simulink library "pixhawk_slib_phm"  (R2017b)
settings: Solver=ode45  StartTime=0.0  StopTime=10.0  RelTol=1e-3
undefined symbols (not defined in the file or in its folder): BatteryFault, Earth, F, FaultParamAPI, Light, LoadFault, MIL, ModelParam_envAltitude, ModelParam_noiseGPSSampTime, ModelParam_noiseLowPassFilterCoeAccel, ModelParam_noiseLowPassFilterCoeGyro, ModelParam_noisePowerIMU, ModelParam_timeSampBaro, Moderate, MotorFault1, PropFault, SensorFault, WGS84, WindFault
libraries: aerolibwind2 x4, aerolibtransform2 x1, simulink x1, aerolibasang x1, aerolibatmos2 x1, aerolibnav x1, aerolibgravity2 x1
(part 1 of 2)
settings Model: Creator=skuznick  LastModifiedBy=uavcs
settings DataIOCC: LimitDataPoints=on  SaveFormat=Array
settings OptimizationCC: BlockReduction=off  BooleanDataType=off  LifeSpan=inf
settings DebuggingCC: SaveWithParameterizedLinksMsg=none  UnderspecifiedInitializationDetection=Classic  MergeDetectMultiDrivingBlocksExec=none  SignalResolutionControl=TryResolveAllWithWarning  AllowSymbolicDim=off  StrictBusMsg=Warning  SFUnexpectedBacktrackingDiag=warning  SFNoUnconditionalDefaultTransitionDiag=warning  SFExecutionAtInitializationDiag=none
settings HardwareCC: ProdBitPerPointer=32  ProdBitPerSizeT=32  ProdBitPerPtrDiffT=32  ProdLargestAtomicFloat=None  ProdIntDivRoundTo=Undefined  ProdEndianess=Unspecified  ProdWordSize=32  ProdHWDeviceType=32-bit Generic  TargetUnknown=on
settings ModelReferenceCC: PropagateSignalLabelsOutOfModel=off
settings CodeAppCC: StateflowObjectComments=on
settings GRTTargetCC: TargetLangStandard=C89/C90 (ANSI)  GeneratePreprocessorConditionals=Disable all
settings ConfigComp: CovMetricSettings=dw  CovHtmlReporting=on  CovSaveCumulativeToWorkspaceVar=on  CovSaveSingleToWorkspaceVar=on  CovExternalEMLEnable=off  CovSFcnEnable=off

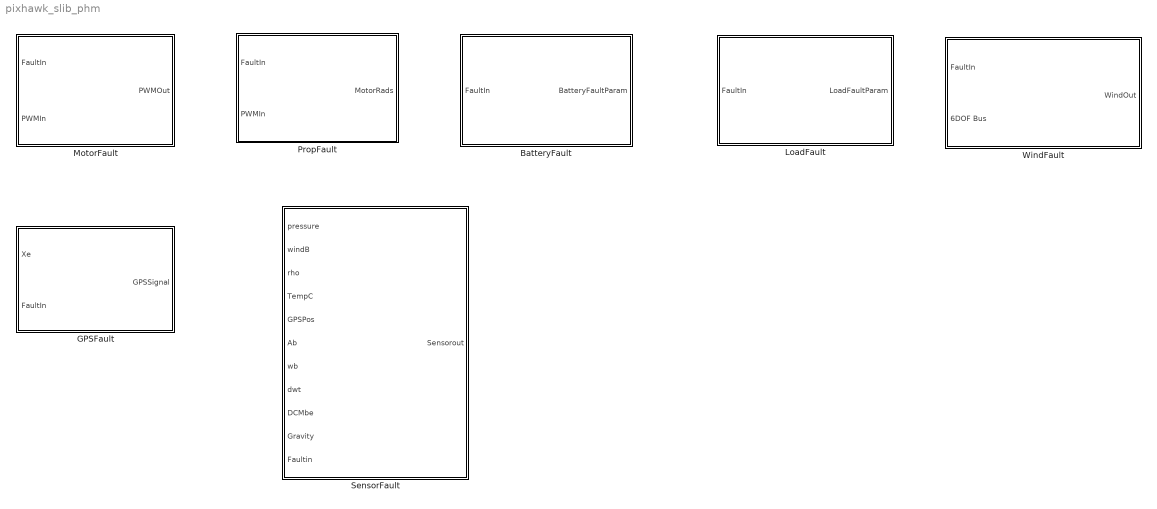
== system pixhawk_slib_phm ==
  BatteryFault : Subsystem  mask{FaultParamStruct=BatteryFault}
      mask prompts: FaultParamStruct "Fault Param Struct"
      mask Help: eval('sharedhelp(''BatteryFault'')');
  GPSFault : Subsystem  mask{FaultParamStruct=SensorFault, ComParamVect=FaultParamAPI}
      mask prompts: FaultParamStruct "Fault Param Struct"; ComParamVect "Common Param Vect"
      mask Help: eval('sharedhelp(''GPSFault'')');
      mask DialogControl ParameterGroupVar Prompt: 参数
  LoadFault : Subsystem  mask{FaultParamStruct=LoadFault}
      mask prompts: FaultParamStruct "Fault Param Struct"
      mask Help: eval('sharedhelp(''LoadFault'')');
  MotorFault : Subsystem  mask{FaultParamStruct=MotorFault1, ComParamVect=FaultParamAPI}
      mask prompts: FaultParamStruct "Fault Param Struct"; ComParamVect "Common Param Vect"
      mask Help: eval('sharedhelp(''MotorFault'')');
  PropFault : Subsystem  mask{FaultParamStruct=PropFault, ComParamVect=FaultParamAPI}
      mask prompts: FaultParamStruct "Fault Param Struct"; ComParamVect "Common Struct Vect"
      mask Help: eval('sharedhelp(''PropFault'')');
  SensorFault : Subsystem  mask{FaultParamStruct=SensorFault, ComParamVect=FaultParamAPI}
      mask prompts: FaultParamStruct "Fault Param Struct"; ComParamVect "Common Param Vect"
      mask Help: eval('sharedhelp(''SensorFault'')');
  WindFault : Subsystem  mask{FaultParamStruct=WindFault, ComParamVect=FaultParamAPI}
      mask prompts: FaultParamStruct "Fault Param Struct"; ComParamVect "Common Param Vect"
      mask Help: eval('sharedhelp(''WindFault'')');

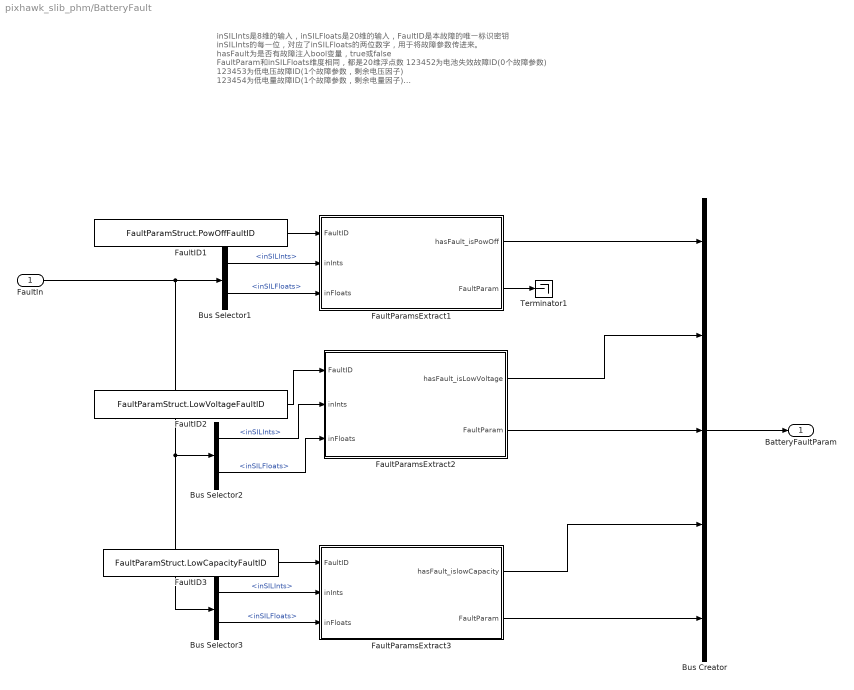
== system pixhawk_slib_phm/BatteryFault ==
  note: inSILInts是8维的输入，inSILFloats是20维的输入，FaultID是本故障的唯一标识密钥
      | inSILInts的每一位，对应了inSILFloats的两位数字，用于将故障参数传进来。
      |
      | hasFault为是否有故障注入bool变量，true或false
      | FaultParam和inSILFloats维度相同，都是20维浮点数
      |
      | 123452为电池失效故障ID(0个故障参数)
      | 123453为低电压故障ID(1个故障参数，剩余电压因子)
      | 123454为低电量故障ID(1个故障参数，剩余电量因子)
      |
      | 注：如果没有新的故障注入进来，FaultParamsExtract会保持上一时刻的值。
  FaultIn : Inport
  Bus Creator : BusCreator  Inputs=5
  Bus Selector1 : BusSelector  OutputSignals=inSILInts,inSILFloats
  Bus Selector2 : BusSelector  OutputSignals=inSILInts,inSILFloats
  Bus Selector3 : BusSelector  OutputSignals=inSILInts,inSILFloats
  FaultID1 : Constant  Value=FaultParamStruct.PowOffFaultID  OutDataTypeStr=int32
  FaultID2 : Constant  Value=FaultParamStruct.LowVoltageFaultID  OutDataTypeStr=int32
  FaultID3 : Constant  Value=FaultParamStruct.LowCapacityFaultID  OutDataTypeStr=int32
  FaultParamsExtract1 : MATLAB Function  TreatAsAtomicUnit=on
  FaultParamsExtract2 : MATLAB Function  TreatAsAtomicUnit=on
  FaultParamsExtract3 : MATLAB Function  TreatAsAtomicUnit=on
  Terminator1 : Terminator
  BatteryFaultParam : Outport  VectorParamsAs1DForOutWhenUnconnected=on
  wires:
  Bus Selector3/2 -> FaultParamsExtract3/3(inFloats)  "<inSILFloats>"
  Bus Selector3/1 -> FaultParamsExtract3/2(inInts)  "<inSILInts>"
  FaultIn/1 -> Bus Selector3/1, Bus Selector2/1, Bus Selector1/1
  Bus Selector1/1 -> FaultParamsExtract1/2(inInts)  "<inSILInts>"
  Bus Selector2/1 -> FaultParamsExtract2/2(inInts)  "<inSILInts>"
  FaultParamsExtract2/2(FaultParam) -> Bus Creator/3
  FaultID2/1 -> FaultParamsExtract2/1(FaultID)
  Bus Selector1/2 -> FaultParamsExtract1/3(inFloats)  "<inSILFloats>"
  FaultID1/1 -> FaultParamsExtract1/1(FaultID)
  FaultID3/1 -> FaultParamsExtract3/1(FaultID)
  Bus Selector2/2 -> FaultParamsExtract2/3(inFloats)  "<inSILFloats>"
  FaultParamsExtract1/2(FaultParam) -> Terminator1/1
  FaultParamsExtract1/1(hasFault_isPowOff) -> Bus Creator/1
  FaultParamsExtract2/1(hasFault_isLowVoltage) -> Bus Creator/2
  Bus Creator/1 -> BatteryFaultParam/1
  FaultParamsExtract3/1(hasFault_islowCapacity) -> Bus Creator/4
  FaultParamsExtract3/2(FaultParam) -> Bus Creator/5

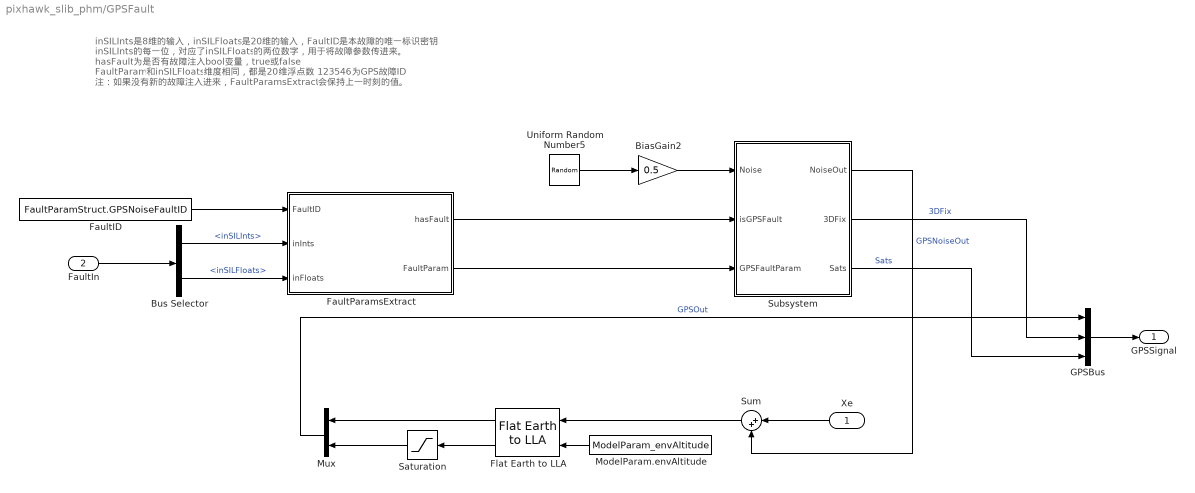
== system pixhawk_slib_phm/GPSFault ==
  note: inSILInts是8维的输入，inSILFloats是20维的输入，FaultID是本故障的唯一标识密钥
      | inSILInts的每一位，对应了inSILFloats的两位数字，用于将故障参数传进来。
      |
      | hasFault为是否有故障注入bool变量，true或false
      | FaultParam和inSILFloats维度相同，都是20维浮点数
      |
      | 123546为GPS故障ID
      |
      | 注：如果没有新的故障注入进来，FaultParamsExtract会保持上一时刻的值。
  Xe : Inport
  FaultIn : Inport  Port=2
  BiasGain2 : Gain  Gain=0.5
  Bus Selector : BusSelector  OutputSignals=inSILInts,inSILFloats
  FaultID : Constant  Value=FaultParamStruct.GPSNoiseFaultID  OutDataTypeStr=int32
  FaultParamsExtract : MATLAB Function  TreatAsAtomicUnit=on
  Flat Earth to LLA : aerolibtransform2/Flat Earth to LLA  units=Metric (MKS)  ptype=Earth (WGS84)  F=1/298.257223563  R=6378137  LL0=ModelParam_GPSLatLong  psi=0
  GPSBus : BusCreator  Inputs=3
  ModelParam.envAltitude : Constant  Value=ModelParam_envAltitude
  Mux : Mux  Inputs=2
  Saturation : Saturate  UpperLimit=100000  LowerLimit=0
  Subsystem : Subsystem
  Sum : Sum  Inputs=|++
  Uniform Random Number5 : UniformRandomNumber  Minimum=[-1,-1,-2]  Maximum=[1,1,2]  Seed=[1452,787,69]  SampleTime=ModelParam_noiseGPSSampTime
  GPSSignal : Outport  VectorParamsAs1DForOutWhenUnconnected=on
  wires:
  FaultParamsExtract/1(hasFault) -> Subsystem/2(isGPSFault)
  FaultParamsExtract/2(FaultParam) -> Subsystem/3(GPSFaultParam)
  Subsystem/3(Sats) -> GPSBus/3  "Sats"
  Saturation/1 -> Mux/2
  Flat Earth to LLA/2 -> Saturation/1
  Uniform Random Number5/1 -> BiasGain2/1
  FaultID/1 -> FaultParamsExtract/1(FaultID)
  BiasGain2/1 -> Subsystem/1(Noise)
  Bus Selector/1 -> FaultParamsExtract/2(inInts)  "<inSILInts>"
  FaultIn/1 -> Bus Selector/1
  Flat Earth to LLA/1 -> Mux/1
  Xe/1 -> Sum/1
  GPSBus/1 -> GPSSignal/1
  Subsystem/2(3DFix) -> GPSBus/2  "3DFix"
  ModelParam.envAltitude/1 -> Flat Earth to LLA/2
  Mux/1 -> GPSBus/1  "GPSOut"
  Subsystem/1(NoiseOut) -> Sum/2  "GPSNoiseOut"
  Bus Selector/2 -> FaultParamsExtract/3(inFloats)  "<inSILFloats>"
  Sum/1 -> Flat Earth to LLA/1

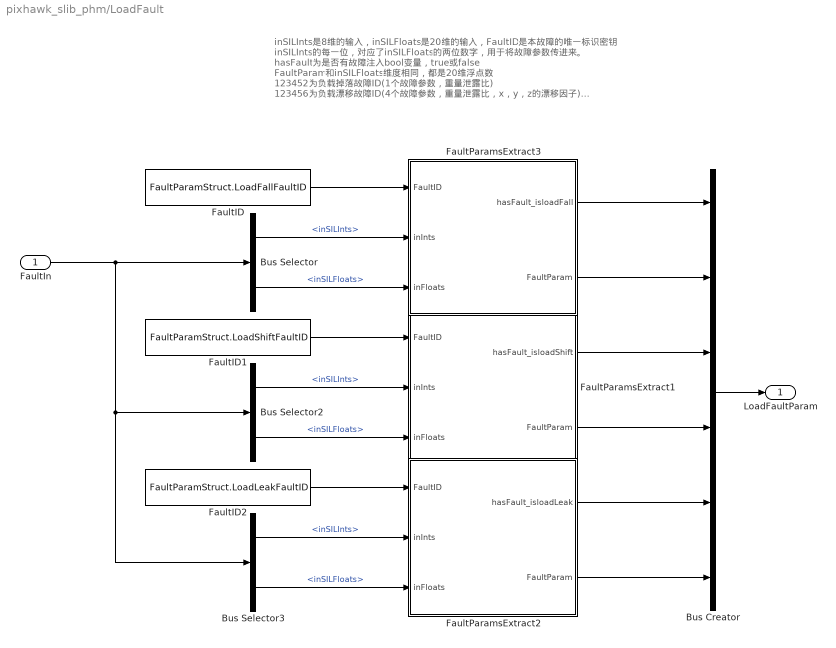
== system pixhawk_slib_phm/LoadFault ==
  note: inSILInts是8维的输入，inSILFloats是20维的输入，FaultID是本故障的唯一标识密钥
      | inSILInts的每一位，对应了inSILFloats的两位数字，用于将故障参数传进来。
      |
      | hasFault为是否有故障注入bool变量，true或false
      | FaultParam和inSILFloats维度相同，都是20维浮点数
      |
      | 123452为负载掉落故障ID(1个故障参数，重量泄露比)
      | 123456为负载漂移故障ID(4个故障参数，重量泄露比，x，y，z的漂移因子)
      | 123457为负载泄露故障ID(2个故障参数，1个重量泄露比，1个泄露因子)
      | 注：如果没有新的故障注入进来，FaultParamsExtract会保持上一时刻的值。
  FaultIn : Inport
  Bus Creator : BusCreator  Inputs=6
  Bus Selector : BusSelector  OutputSignals=inSILInts,inSILFloats
  Bus Selector2 : BusSelector  OutputSignals=inSILInts,inSILFloats
  Bus Selector3 : BusSelector  OutputSignals=inSILInts,inSILFloats
  FaultID : Constant  Value=FaultParamStruct.LoadFallFaultID  OutDataTypeStr=int32
  FaultID1 : Constant  Value=FaultParamStruct.LoadShiftFaultID  OutDataTypeStr=int32
  FaultID2 : Constant  Value=FaultParamStruct.LoadLeakFaultID  OutDataTypeStr=int32
  FaultParamsExtract1 : MATLAB Function  TreatAsAtomicUnit=on
  FaultParamsExtract2 : MATLAB Function  TreatAsAtomicUnit=on
  FaultParamsExtract3 : MATLAB Function  TreatAsAtomicUnit=on
  LoadFaultParam : Outport  VectorParamsAs1DForOutWhenUnconnected=on
  wires:
  FaultIn/1 -> Bus Selector3/1, Bus Selector2/1, Bus Selector/1
  Bus Selector3/2 -> FaultParamsExtract2/3(inFloats)  "<inSILFloats>"
  Bus Selector/1 -> FaultParamsExtract3/2(inInts)  "<inSILInts>"
  Bus Selector2/2 -> FaultParamsExtract1/3(inFloats)  "<inSILFloats>"
  Bus Selector3/1 -> FaultParamsExtract2/2(inInts)  "<inSILInts>"
  Bus Selector2/1 -> FaultParamsExtract1/2(inInts)  "<inSILInts>"
  Bus Selector/2 -> FaultParamsExtract3/3(inFloats)  "<inSILFloats>"
  FaultID/1 -> FaultParamsExtract3/1(FaultID)
  FaultID2/1 -> FaultParamsExtract2/1(FaultID)
  FaultID1/1 -> FaultParamsExtract1/1(FaultID)
  FaultParamsExtract3/1(hasFault_isloadFall) -> Bus Creator/1
  FaultParamsExtract3/2(FaultParam) -> Bus Creator/2
  FaultParamsExtract1/1(hasFault_isloadShift) -> Bus Creator/3
  FaultParamsExtract1/2(FaultParam) -> Bus Creator/4
  FaultParamsExtract2/1(hasFault_isloadLeak) -> Bus Creator/5
  FaultParamsExtract2/2(FaultParam) -> Bus Creator/6
  Bus Creator/1 -> LoadFaultParam/1

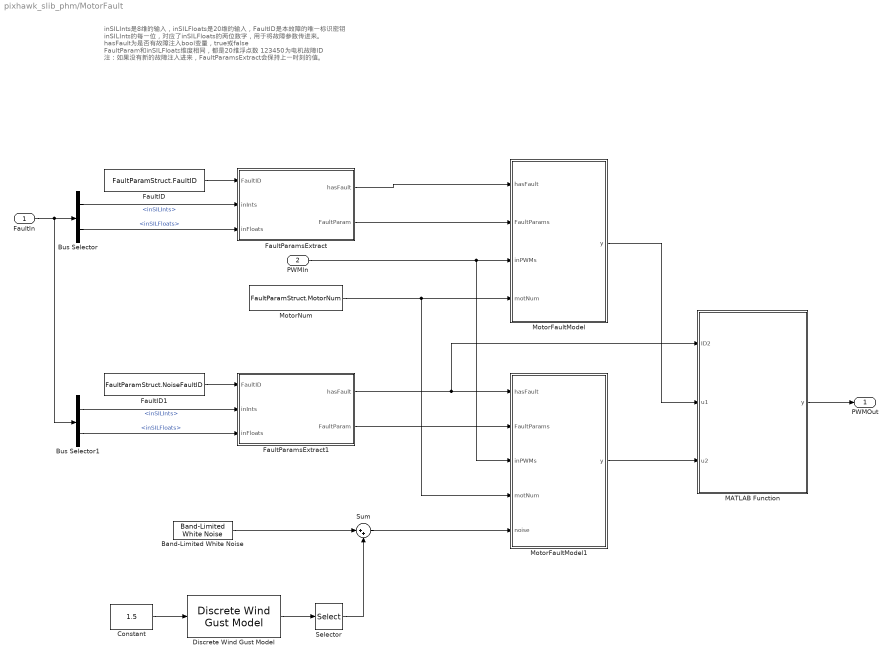
== system pixhawk_slib_phm/MotorFault ==
  note: inSILInts是8维的输入，inSILFloats是20维的输入，FaultID是本故障的唯一标识密钥
      | inSILInts的每一位，对应了inSILFloats的两位数字，用于将故障参数传进来。
      |
      | hasFault为是否有故障注入bool变量，true或false
      | FaultParam和inSILFloats维度相同，都是20维浮点数
      |
      | 123450为电机故障ID
      |
      | 注：如果没有新的故障注入进来，FaultParamsExtract会保持上一时刻的值。
  FaultIn : Inport
  PWMIn : Inport  Port=2
  Band-Limited White Noise : simulink/Sources/Band-Limited White Noise  Cov=[1]  Ts=0.1  seed=[23341]
  Bus Selector : BusSelector  OutputSignals=inSILInts,inSILFloats
  Bus Selector1 : BusSelector  OutputSignals=inSILInts,inSILFloats
  Constant : Constant  Value=1.5
  Discrete Wind Gust Model : aerolibwind2/Discrete Wind Gust Model  units=Metric (MKS)  Gx=on  Gy=on  Gz=on  t_0=ComParamVect.FaultInParams(3)  d_m=[120 120 80]  v_m=[3.5 3.5 3.0]
  FaultID : Constant  Value=FaultParamStruct.FaultID  OutDataTypeStr=int32
  FaultID1 : Constant  Value=FaultParamStruct.NoiseFaultID  OutDataTypeStr=int32
  FaultParamsExtract : MATLAB Function  TreatAsAtomicUnit=on
  FaultParamsExtract1 : MATLAB Function  TreatAsAtomicUnit=on
  MATLAB Function : MATLAB Function  TreatAsAtomicUnit=on
  MotorFaultModel : MATLAB Function  TreatAsAtomicUnit=on
  MotorFaultModel1 : MATLAB Function  TreatAsAtomicUnit=on
  MotorNum : Constant  Value=FaultParamStruct.MotorNum  OutDataTypeStr=int32
  Selector : Selector  InputPortWidth=3  IndexOptions=Index vector (dialog)  Indices=[1]  OutputSizes=1
  Sum : Sum  Inputs=|++
  PWMOut : Outport  VectorParamsAs1DForOutWhenUnconnected=on
  wires:
  FaultIn/1 -> Bus Selector1/1, Bus Selector/1
  FaultParamsExtract/2(FaultParam) -> MotorFaultModel/2(FaultParams)
  FaultParamsExtract/1(hasFault) -> MotorFaultModel/1(hasFault)
  PWMIn/1 -> MotorFaultModel1/3(inPWMs), MotorFaultModel/3(inPWMs)
  FaultID/1 -> FaultParamsExtract/1(FaultID)
  MotorFaultModel/1(y) -> MATLAB Function/2(u1)
  Bus Selector/2 -> FaultParamsExtract/3(inFloats)  "<inSILFloats>"
  Constant/1 -> Discrete Wind Gust Model/1
  Selector/1 -> Sum/2
  Sum/1 -> MotorFaultModel1/5(noise)
  Discrete Wind Gust Model/1 -> Selector/1
  Band-Limited White Noise/1 -> Sum/1
  Bus Selector/1 -> FaultParamsExtract/2(inInts)  "<inSILInts>"
  MotorNum/1 -> MotorFaultModel1/4(motNum), MotorFaultModel/4(motNum)
  Bus Selector1/1 -> FaultParamsExtract1/2(inInts)  "<inSILInts>"
  Bus Selector1/2 -> FaultParamsExtract1/3(inFloats)  "<inSILFloats>"
  FaultParamsExtract1/1(hasFault) -> MATLAB Function/1(ID2), MotorFaultModel1/1(hasFault)
  FaultParamsExtract1/2(FaultParam) -> MotorFaultModel1/2(FaultParams)
  FaultID1/1 -> FaultParamsExtract1/1(FaultID)
  MotorFaultModel1/1(y) -> MATLAB Function/3(u2)
  MATLAB Function/1(y) -> PWMOut/1

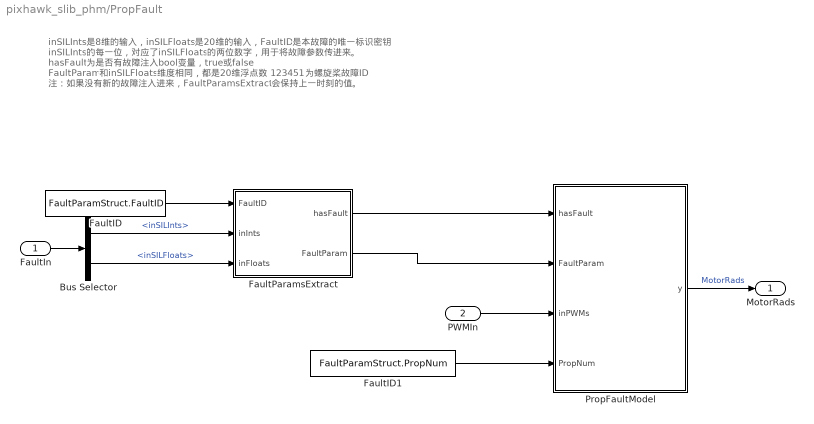
== system pixhawk_slib_phm/PropFault ==
  note: inSILInts是8维的输入，inSILFloats是20维的输入，FaultID是本故障的唯一标识密钥
      | inSILInts的每一位，对应了inSILFloats的两位数字，用于将故障参数传进来。
      |
      | hasFault为是否有故障注入bool变量，true或false
      | FaultParam和inSILFloats维度相同，都是20维浮点数
      |
      | 123451为螺旋桨故障ID
      | 注：如果没有新的故障注入进来，FaultParamsExtract会保持上一时刻的值。
  FaultIn : Inport
  PWMIn : Inport  Port=2
  Bus Selector : BusSelector  OutputSignals=inSILInts,inSILFloats
  FaultID : Constant  Value=FaultParamStruct.FaultID  OutDataTypeStr=int32
  FaultID1 : Constant  Value=FaultParamStruct.PropNum  OutDataTypeStr=int32
  FaultParamsExtract : MATLAB Function  TreatAsAtomicUnit=on
  PropFaultModel : MATLAB Function  TreatAsAtomicUnit=on
  MotorRads : Outport
  wires:
  FaultParamsExtract/1(hasFault) -> PropFaultModel/1(hasFault)
  Bus Selector/2 -> FaultParamsExtract/3(inFloats)  "<inSILFloats>"
  FaultID/1 -> FaultParamsExtract/1(FaultID)
  Bus Selector/1 -> FaultParamsExtract/2(inInts)  "<inSILInts>"
  FaultParamsExtract/2(FaultParam) -> PropFaultModel/2(FaultParam)
  PWMIn/1 -> PropFaultModel/3(inPWMs)
  PropFaultModel/1(y) -> MotorRads/1  "MotorRads"
  FaultIn/1 -> Bus Selector/1
  FaultID1/1 -> PropFaultModel/4(PropNum)

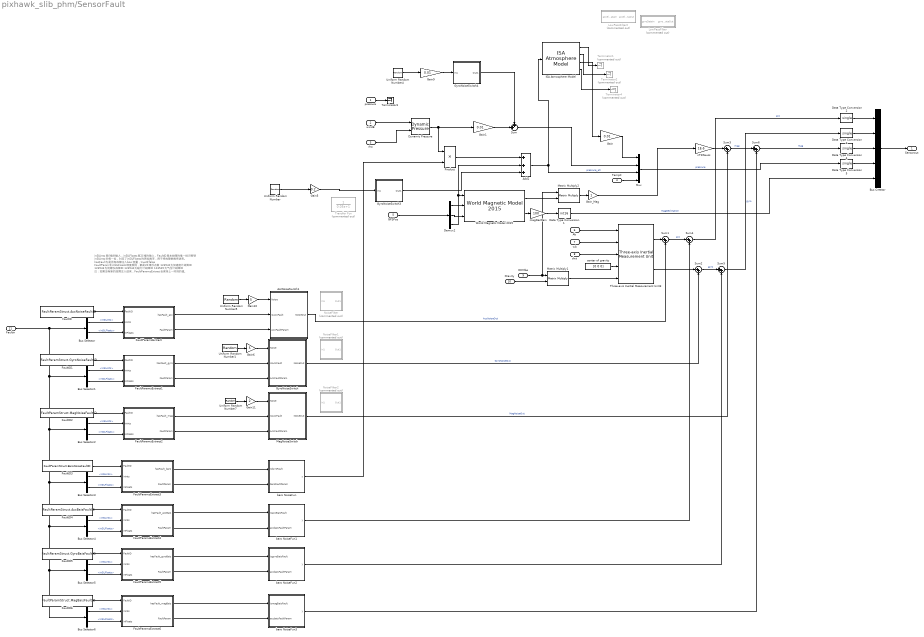
== system pixhawk_slib_phm/SensorFault ==
  note: inSILInts是8维的输入，inSILFloats是20维的输入，FaultID是本故障的唯一标识密钥
      | inSILInts的每一位，对应了inSILFloats的两位数字，用于将故障参数传进来。
      |
      | hasFault为是否有故障注入bool变量，true或false
      | FaultParam和inSILFloats维度相同，都是20维浮点数
      |
      | 123542为加速度计故障ID
      | 123543为陀螺仪故障ID
      | 123544为磁力计故障ID
      | 123545为气压计故障ID
      | 注：如果没有新的故障注入进来，FaultParamsExtract会保持上一时刻的值。
  pressure : Inport
  windB : Inport  Port=2
  rho : Inport  Port=3
  TempC : Inport  Port=4
  GPSPos : Inport  Port=5
  Ab : Inport  Port=6
  wb : Inport  Port=7
  dwt : Inport  Port=8
  DCMbe : Inport  Port=9
  Gravity : Inport  Port=10
  Faultin : Inport  Port=11
  AccNoiseSwitch1 : Subsystem
  Add2 : Sum  Inputs=+++
  Bus Creator : BusCreator  Inputs=5
  Bus Selector{,1..6} (7 alike) : BusSelector  OutputSignals=inSILInts,inSILFloats
  Data Type Conversion1 : DataTypeConversion  OutDataTypeStr=int16
  Data Type Conversion{2..5} (4 alike) : DataTypeConversion  OutDataTypeStr=single
  Demux2 : Demux  Outputs=3
  Dynamic Pressure : aerolibasang/Dynamic Pressure
  FaultID : Constant  Value=FaultParamStruct.AccNoiseFaultID  OutDataTypeStr=int32
  FaultID1 : Constant  Value=FaultParamStruct.GyroNoiseFaultID  OutDataTypeStr=int32
  FaultID2 : Constant  Value=FaultParamStruct.MagNoiseFaultID  OutDataTypeStr=int32
  FaultID3 : Constant  Value=FaultParamStruct.BaroNoiseFaultID  OutDataTypeStr=int32
  FaultID4 : Constant  Value=FaultParamStruct.AccBaisFaultID  OutDataTypeStr=int32
  FaultID5 : Constant  Value=FaultParamStruct.GyroBaisFaultID  OutDataTypeStr=int32
  FaultID6 : Constant  Value=FaultParamStruct.MagBaisFaultID  OutDataTypeStr=int32
  FaultParamsExtract : MATLAB Function  TreatAsAtomicUnit=on
  FaultParamsExtract1 : MATLAB Function  TreatAsAtomicUnit=on
  FaultParamsExtract2 : MATLAB Function  TreatAsAtomicUnit=on
  FaultParamsExtract3 : MATLAB Function  TreatAsAtomicUnit=on
  FaultParamsExtract4 : MATLAB Function  TreatAsAtomicUnit=on
  FaultParamsExtract5 : MATLAB Function  TreatAsAtomicUnit=on
  FaultParamsExtract6 : MATLAB Function  TreatAsAtomicUnit=on
  Gain : Gain  Gain=0.01
  Gain1 : Gain  Gain=0.01
  Gain10 : Gain  Gain=5
  Gain11 : Gain  Gain=2
  Gain5 : Gain  Gain=0.2
  Gain6 : Gain  Gain=5
  Gain9 : Gain  Gain=0.01
  Gain_Mag : Gain
  GyroNoiseSwitch : Subsystem
  GyroNoiseSwitch3 : Subsystem
  GyroNoiseSwitch4 : Subsystem
  ISA Atmosphere Model : aerolibatmos2/ISA Atmosphere Model  custom=off  g=9.80665  gamma=1.4  R=287.0531  L=0.0065  h_trop=11000  h_strat=20000  rho0=1.225  P0=101325  T0=288.15  h0=0
  LowPassFilter : Subsystem  Commented=on
  LowPassFilter2 : Subsystem  Commented=on
  MagNoiseSwitch : Subsystem
  Matrix Multiply1 : Product  Multiplication=Matrix(*)
  Matrix Multiply2 : Product  Multiplication=Matrix(*)
  Mux : Mux
  NoiseFilter : Subsystem  Commented=on
  NoiseFilter1 : Subsystem  Commented=on
  NoiseFilter2 : Subsystem  Commented=on
  Product : Product
  Sum : Sum  Inputs=++|
  Sum{1..6} (6 alike) : Sum  Inputs=|++
  Terminator1 : Terminator  Commented=on
  Terminator2 : Terminator  Commented=on
  Terminator3 : Terminator
  Terminator4 : Terminator  Commented=on
  Three-axis Inertial Measurement Unit3 : aerolibnav/Three-axis Inertial Measurement Unit  units=Metric (MKS)  imu=[0 0 0]  i_Ts=0  dtype_a=on  w_a=ComParamVect.FaultInParams(1)  z_a=ComParamVect.FaultInParams(2)  a_sf_cc=[1 0 0; 0 1 0; 0 0 1]  a_bias=[ComParamVect.FaultInParams(3) ComParamVect.FaultInParams(4) ComParamVect.FaultInParams(5)]  a_sat="[-160  -160  -160 160 160 160]"  dtype_g=on  w_g=ComParamVect.FaultInParams(6)  z_g=ComParamVect.FaultInParams(7)  g_sf_cc=[1 0 0; 0 1 0; 0 0 1]  g_bias=[ComParamVect.FaultInParams(8) ComParamVect.FaultInParams(9) ComParamVect.FaultInParams(10)]  g_sens=[ComParamVect.FaultInParams(11) ComParamVect.FaultInParams(12) ComParamVect.FaultInParams(13)]  g_sat="[-4.36  -4.36  -4.36 4.36 4.36 4.36]"  i_rand=off  i_seeds=[23093 23094 23095 23096 23097 23098]  i_pow=ModelParam_noisePowerIMU*[0.0000005 0.0000005 0.0000005 0.000000002 0.000000002 0.000000002]
  Transfer Fcn : TransferFcn  Commented=on  Denominator=[0.05 1]
  Uniform Random Number : UniformRandomNumber  Minimum=-2  Maximum=2  Seed=15634  SampleTime=ModelParam_timeSampBaro
  Uniform Random Number1 : UniformRandomNumber  Minimum=-[0.01,0.01,0.01]  Maximum=[0.01,0.01,0.01]  Seed=[3243,44556,2334343]  SampleTime=0.003
  Uniform Random Number4 : UniformRandomNumber  Seed=25634  SampleTime=0.01
  Uniform Random Number5 : UniformRandomNumber  Minimum=-[0.1,0.1,0.2]  Maximum=[0.1,0.1,0.2]  Seed=[12233,645554,678766]  SampleTime=0.003
  Uniform Random Number7 : UniformRandomNumber  Minimum=-[0.01,0.01,0.01]  Maximum=[0.01,0.01,0.01]  Seed=[45465,454534,1234232]  SampleTime=0.003
  World Magnetic Model 2015 : aerolibgravity2/World Magnetic Model 2015  units=Metric (MKS)  time_in=off  month=November  day=3  year=2017  action=Error  h_out=off  dec_out=on  inc_out=off  ti_out=off
      settings: SourceProductBaseCode=AE
  baro NoiseFun : MATLAB Function  TreatAsAtomicUnit=on
  baro NoiseFun1 : MATLAB Function  TreatAsAtomicUnit=on
  baro NoiseFun2 : MATLAB Function  TreatAsAtomicUnit=on
  baro NoiseFun3 : MATLAB Function  TreatAsAtomicUnit=on
  center of gravity : Constant  Value=[0 0 0]
  magDecGain : Gain  Gain=100
  nT2Gauss : Gain  Gain=1E-5
  Sensorout : Outport  VectorParamsAs1DForOutWhenUnconnected=on
  wires:
  FaultParamsExtract3/2(FaultParam) -> baro NoiseFun/2(baroFaultParam)
  Gain9/1 -> GyroNoiseSwitch4/1(In1)
  Matrix Multiply1/1 -> Three-axis Inertial Measurement Unit3/5
  Three-axis Inertial Measurement Unit3/1 -> Sum1/1
  FaultParamsExtract1/1(hasFault_gyro) -> GyroNoiseSwitch/2(isAccFault)
  FaultParamsExtract1/2(FaultParam) -> GyroNoiseSwitch/3(AccFaultParam)
  FaultParamsExtract/1(hasFault_acc) -> AccNoiseSwitch1/2(isAccFault)
  Bus Selector3/1 -> FaultParamsExtract3/2(inInts)  "<inSILInts>"
  Mux/1 -> Data Type Conversion5/1  "pressure"
  FaultID/1 -> FaultParamsExtract/1(FaultID)
  Sum/1 -> Mux/2
  Add2/1 -> ISA Atmosphere Model/1, Mux/3  "pressure_alt"
  TempC/1 -> Mux/4
  Gain11/1 -> MagNoiseSwitch/1(Noise)
  nT2Gauss/1 -> Sum3/1
  center of gravity/1 -> Three-axis Inertial Measurement Unit3/4
  Gravity/1 -> Matrix Multiply1/2
  Bus Selector1/2 -> FaultParamsExtract1/3(inFloats)  "<inSILFloats>"
  FaultID2/1 -> FaultParamsExtract2/1(FaultID)
  World Magnetic Model 2015/1 -> Matrix Multiply2/2
  Bus Selector3/2 -> FaultParamsExtract3/3(inFloats)  "<inSILFloats>"
  magDecGain/1 -> Data Type Conversion1/1
  DCMbe/1 -> Matrix Multiply2/1, Matrix Multiply1/1
  Three-axis Inertial Measurement Unit3/2 -> Sum2/1
  Gain_Mag/1 -> nT2Gauss/1
  Bus Selector1/1 -> FaultParamsExtract1/2(inInts)  "<inSILInts>"
  Gain6/1 -> GyroNoiseSwitch/1(Noise)
  ISA Atmosphere Model/3 -> Gain/1
  Gain1/1 -> Sum/2
  Bus Selector/2 -> FaultParamsExtract/3(inFloats)  "<inSILFloats>"
  FaultParamsExtract3/1(hasFault_baro) -> baro NoiseFun/1(isbyroFault)
  Uniform Random Number1/1 -> Gain6/1
  FaultID1/1 -> FaultParamsExtract1/1(FaultID)
  baro NoiseFun/1(y) -> Product/2
  GyroNoiseSwitch/1(NoiseOut) -> Sum2/2  "GyroNoiseOut"
  ISA Atmosphere Model/1 -> Terminator1/1
  Gain/1 -> Mux/1
  pressure/1 -> Terminator3/1
  Demux2/1 -> World Magnetic Model 2015/2
  Bus Selector2/1 -> FaultParamsExtract2/2(inInts)  "<inSILInts>"
  Uniform Random Number4/1 -> Gain9/1
  GyroNoiseSwitch4/1(Out1) -> Sum/1
  ISA Atmosphere Model/2 -> Terminator2/1
  windB/1 -> Dynamic Pressure/1
  FaultID3/1 -> FaultParamsExtract3/1(FaultID)
  GPSPos/1 -> Demux2/1
  Uniform Random Number/1 -> Gain5/1
  Bus Selector/1 -> FaultParamsExtract/2(inInts)  "<inSILInts>"
  dwt/1 -> Three-axis Inertial Measurement Unit3/3
  FaultParamsExtract2/2(FaultParam) -> MagNoiseSwitch/3(AccFaultParam)
  World Magnetic Model 2015/2 -> magDecGain/1
  GyroNoiseSwitch3/1(Out1) -> Add2/3
  Faultin/1 -> Bus Selector3/1, Bus Selector5/1, Bus Selector6/1, Bus Selector4/1, Bus Selector2/1, Bus Selector1/1, Bus Selector/1
  Demux2/3 -> World Magnetic Model 2015/1, Add2/2
  Bus Selector2/2 -> FaultParamsExtract2/3(inFloats)  "<inSILFloats>"
  MagNoiseSwitch/1(NoiseOut) -> Sum3/2  "MagNoiseOut"
  Gain10/1 -> AccNoiseSwitch1/1(Noise)
  Dynamic Pressure/1 -> Gain1/1, Product/1
  Uniform Random Number7/1 -> Gain11/1
  Matrix Multiply2/1 -> Gain_Mag/1
  Uniform Random Number5/1 -> Gain10/1
  Product/1 -> Add2/1
  ISA Atmosphere Model/4 -> Terminator4/1
  FaultParamsExtract2/1(hasFault_mag) -> MagNoiseSwitch/2(isAccFault)
  Gain5/1 -> GyroNoiseSwitch3/1(In1)
  Demux2/2 -> World Magnetic Model 2015/3
  FaultParamsExtract/2(FaultParam) -> AccNoiseSwitch1/3(AccFaultParam)
  rho/1 -> Dynamic Pressure/2
  Data Type Conversion1/1 -> Bus Creator/5  "MagDeclination"
  Bus Creator/1 -> Sensorout/1
  Data Type Conversion2/1 -> Bus Creator/1
  Data Type Conversion3/1 -> Bus Creator/2
  Data Type Conversion4/1 -> Bus Creator/3
  Data Type Conversion5/1 -> Bus Creator/4
  Ab/1 -> Three-axis Inertial Measurement Unit3/1
  wb/1 -> Three-axis Inertial Measurement Unit3/2
  AccNoiseSwitch1/1(NoiseOut) -> Sum1/2  "AccNoiseOut"
  FaultID4/1 -> FaultParamsExtract4/1(FaultID)
  Bus Selector4/1 -> FaultParamsExtract4/2(inInts)  "<inSILInts>"
  Bus Selector4/2 -> FaultParamsExtract4/3(inFloats)  "<inSILFloats>"
  FaultParamsExtract4/1(hasFault_accBais) -> baro NoiseFun1/1(isaccBaisFault)
  FaultParamsExtract4/2(FaultParam) -> baro NoiseFun1/2(accbaisFaultParam)
  Sum1/1 -> Sum4/1  "acc"
  Sum4/1 -> Data Type Conversion2/1  "acc"
  baro NoiseFun1/1(y) -> Sum4/2
  FaultParamsExtract5/1(hasFault_gyroBais) -> baro NoiseFun2/1(isgyroBaisFault)
  Bus Selector5/2 -> FaultParamsExtract5/3(inFloats)  "<inSILFloats>"
  Bus Selector5/1 -> FaultParamsExtract5/2(inInts)  "<inSILInts>"
  FaultID5/1 -> FaultParamsExtract5/1(FaultID)
  FaultParamsExtract5/2(FaultParam) -> baro NoiseFun2/2(accbaisFaultParam)
  FaultID6/1 -> FaultParamsExtract6/1(FaultID)
  FaultParamsExtract6/2(FaultParam) -> baro NoiseFun3/2(accbaisFaultParam)
  Bus Selector6/2 -> FaultParamsExtract6/3(inFloats)  "<inSILFloats>"
  FaultParamsExtract6/1(hasFault_magBais) -> baro NoiseFun3/1(ismagBaisFault)
  Bus Selector6/1 -> FaultParamsExtract6/2(inInts)  "<inSILInts>"
  Sum2/1 -> Sum5/1  "gyro"
  Sum5/1 -> Data Type Conversion3/1  "gyro"
  baro NoiseFun2/1(y) -> Sum5/2
  Sum3/1 -> Sum6/1  "mag"
  baro NoiseFun3/1(y) -> Sum6/2
  Sum6/1 -> Data Type Conversion4/1  "mag"

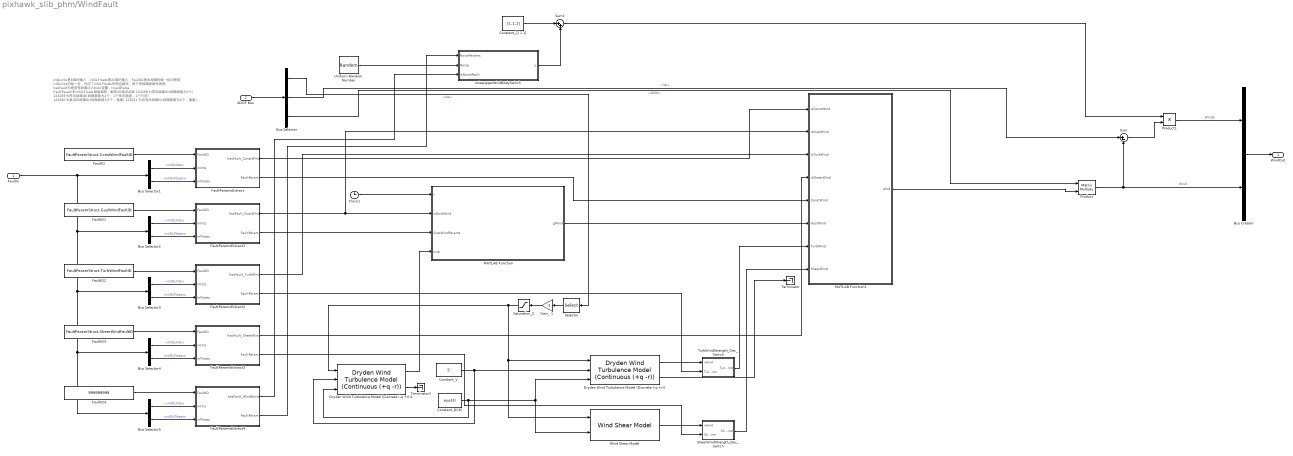
== system pixhawk_slib_phm/WindFault ==
  note: inSILInts是8维的输入，inSILFloats是20维的输入，FaultID是本故障的唯一标识密钥
      | inSILInts的每一位，对应了inSILFloats的两位数字，用于将故障参数传进来。
      |
      | hasFault为是否有故障注入bool变量，true或false
      | FaultParam和inSILFloats维度相同，都是20维浮点数
      |
      | 123458为常风故障ID(故障参数为3个)
      | 123459为阵风故障ID(故障参数为2个，1个阵风强度，1个方向)
      | 123540为紊流风故障ID(故障参数为1个，强度)
      | 123541为切向风故障ID(故障参数为1个，强度)
      |
      | 注：如果没有新的故障注入进来，FaultParamsExtract会保持上一时刻的值。
  FaultIn : Inport
  6DOF Bus : Inport  Port=2
  Bus Creator : BusCreator  Inputs=2
  Bus Selector : BusSelector  OutputSignals=Xe,Vb,DCM
  Bus Selector{1..5} (5 alike) : BusSelector  OutputSignals=inSILInts,inSILFloats
  Clock1 : Clock
  Constant_DCM : Constant  Value=eye(3)
  Constant_V : Constant  Value=5
  Constant_[1 1 1] : Constant  Value=[1,1,1]  VectorParams1D=off
  Dryden Wind Turbulence Model (Discrete (-q +r)) : aerolibwind2/Dryden Wind Turbulence Model  (Continuous (+q -r))  units=Metric (MKS)  spec=MIL-F-8785C  model=Discrete Dryden (-q +r)  W20=3  Wdeg=1  TurbProb=10^-3 - Moderate  L_high=533.4  Wingspan=1  ts=ModelParam_timeSampTurbWind  Seed=[23341 23342 23343 23344]  T_on=on
  Dryden Wind Turbulence Model (Discrete (-q +r))1 : aerolibwind2/Dryden Wind Turbulence Model  (Continuous (+q -r))  units=Metric (MKS)  spec=MIL-F-8785C  model=Discrete Dryden (-q +r)  W20=2  Wdeg=1  TurbProb=10^-2 - Light  L_high=533.4  Wingspan=1  ts=ModelParam_timeSampTurbWind  Seed=[23301 23542 82443 33344]  T_on=on
  FaultID : Constant  Value=FaultParamStruct.ConstWindFaultID  OutDataTypeStr=int32
  FaultID1 : Constant  Value=FaultParamStruct.GustWindFaultID  OutDataTypeStr=int32
  FaultID2 : Constant  Value=FaultParamStruct.TurbWindFaultID  OutDataTypeStr=int32
  FaultID3 : Constant  Value=FaultParamStruct.SheerWindFaultID  OutDataTypeStr=int32
  FaultID4 : Constant  Value=999999999  OutDataTypeStr=int32
  FaultParamsExtract : MATLAB Function  TreatAsAtomicUnit=on
  FaultParamsExtract1 : MATLAB Function  TreatAsAtomicUnit=on
  FaultParamsExtract2 : MATLAB Function  TreatAsAtomicUnit=on
  FaultParamsExtract3 : MATLAB Function  TreatAsAtomicUnit=on
  FaultParamsExtract4 : MATLAB Function  TreatAsAtomicUnit=on
  Gain_-1 : Gain  Gain=-1
  MATLAB Function : MATLAB Function  TreatAsAtomicUnit=on
  MATLAB Function1 : MATLAB Function  TreatAsAtomicUnit=on
  Product : Product  Multiplication=Matrix(*)
  Product1 : Product
  Saturation_2 : Saturate  UpperLimit=10000  LowerLimit=0
  Selector : Selector  InputPortWidth=3  IndexOptions=Index vector (dialog)  Indices=[3]  OutputSizes=1
  SheerWindStrength_Dec_Switch : MATLAB Function  TreatAsAtomicUnit=on
  Sum : Sum  Inputs=|+-
  Sum1 : Sum  Inputs=|++
  Terminator : Terminator
  Terminator1 : Terminator
  TurbWindStrength_Dec_Switch : MATLAB Function  TreatAsAtomicUnit=on
  Uniform Random Number : UniformRandomNumber  Minimum=[-1,-1,-0.5]  Maximum=[1,1,0.5]  Seed=[564565,6846798,46545]  SampleTime=0.003
  Wind Shear Model : aerolibwind2/Wind Shear Model  units=Metric (MKS)  phase=Category C - Terminal Flight Phase  W_20=3  Wdeg=1
  noiseUpperWindBodySwitch : MATLAB Function  TreatAsAtomicUnit=on
  WindOut : Outport  VectorParamsAs1DForOutWhenUnconnected=on
  wires:
  Product/1 -> Bus Creator/2, Sum/2  "Wind"
  Constant_DCM/1 -> Dryden Wind Turbulence Model (Discrete (-q +r))/3, Wind Shear Model/2, Dryden Wind Turbulence Model (Discrete (-q +r))1/3
  Clock1/1 -> MATLAB Function/1(t)
  FaultParamsExtract2/2(FaultParam) -> TurbWindStrength_Dec_Switch/2(TurbWindParams)
  FaultID1/1 -> FaultParamsExtract1/1(FaultID)
  FaultIn/1 -> Bus Selector5/1, Bus Selector4/1, Bus Selector3/1, Bus Selector2/1, Bus Selector1/1
  Bus Selector2/2 -> FaultParamsExtract1/3(inFloats)  "<inSILFloats>"
  Bus Selector1/2 -> FaultParamsExtract/3(inFloats)  "<inSILFloats>"
  MATLAB Function/1(gWind) -> MATLAB Function1/6(GustWind)
  FaultID2/1 -> FaultParamsExtract2/1(FaultID)
  Sum1/1 -> Product1/1
  FaultID4/1 -> FaultParamsExtract4/1(FaultID)
  Uniform Random Number/1 -> noiseUpperWindBodySwitch/2(Noise)
  Bus Selector1/1 -> FaultParamsExtract/2(inInts)  "<inSILInts>"
  FaultParamsExtract/2(FaultParam) -> MATLAB Function1/5(ConstWind)
  FaultParamsExtract4/1(hasFault_WindNoise) -> noiseUpperWindBodySwitch/3(isNoiseFault)
  Dryden Wind Turbulence Model (Discrete (-q +r))1/1 -> MATLAB Function/4(turb)
  Bus Selector5/2 -> FaultParamsExtract4/3(inFloats)  "<inSILFloats>"
  noiseUpperWindBodySwitch/1(y) -> Sum1/2
  FaultParamsExtract1/1(hasFault_GustWind) -> MATLAB Function/2(isGustWind), MATLAB Function1/2(isGustWind)
  Dryden Wind Turbulence Model (Discrete (-q +r))/2 -> Terminator/1
  Bus Selector3/2 -> FaultParamsExtract2/3(inFloats)  "<inSILFloats>"
  FaultParamsExtract3/1(hasFault_SheerWind) -> MATLAB Function1/4(isSheerWind)
  SheerWindStrength_Dec_Switch/1(SheerWind) -> MATLAB Function1/8(SheerWind)
  Bus Selector4/2 -> FaultParamsExtract3/3(inFloats)  "<inSILFloats>"
  Dryden Wind Turbulence Model (Discrete (-q +r))/1 -> TurbWindStrength_Dec_Switch/1(vwind)
  Bus Selector3/1 -> FaultParamsExtract2/2(inInts)  "<inSILInts>"
  Sum/1 -> Product1/2
  FaultParamsExtract3/2(FaultParam) -> SheerWindStrength_Dec_Switch/2(SheerWindParams)
  FaultID/1 -> FaultParamsExtract/1(FaultID)
  Wind Shear Model/1 -> SheerWindStrength_Dec_Switch/1(vwind)
  FaultParamsExtract4/2(FaultParam) -> noiseUpperWindBodySwitch/1(NoiseParams)
  Dryden Wind Turbulence Model (Discrete (-q +r))1/2 -> Terminator1/1
  Constant_[1 1 1]/1 -> Sum1/1
  Constant_V/1 -> Dryden Wind Turbulence Model (Discrete (-q +r))1/2, Dryden Wind Turbulence Model (Discrete (-q +r))/2
  MATLAB Function1/1(wind) -> Product/2
  FaultParamsExtract2/1(hasFault_TurbWind) -> MATLAB Function1/3(isTurbWind)
  FaultParamsExtract1/2(FaultParam) -> MATLAB Function/3(GustWindParams)
  TurbWindStrength_Dec_Switch/1(TurbWind) -> MATLAB Function1/7(TurbWind)
  Bus Selector4/1 -> FaultParamsExtract3/2(inInts)  "<inSILInts>"
  FaultID3/1 -> FaultParamsExtract3/1(FaultID)
  FaultParamsExtract/1(hasFault_ConstWind) -> MATLAB Function1/1(isConstWind)
  Bus Selector2/1 -> FaultParamsExtract1/2(inInts)  "<inSILInts>"
  Bus Selector5/1 -> FaultParamsExtract4/2(inInts)  "<inSILInts>"
  Bus Selector/3 -> Product/1  "<DCM>"
  Bus Selector/2 -> Sum/1  "<Vb>"
  6DOF Bus/1 -> Bus Selector/1
  Selector/1 -> Gain_-1/1
  Gain_-1/1 -> Saturation_2/1
  Bus Selector/1 -> Selector/1  "<Xe>"
  Saturation_2/1 -> Wind Shear Model/1, Dryden Wind Turbulence Model (Discrete (-q +r))/1, Dryden Wind Turbulence Model (Discrete (-q +r))1/1
  Product1/1 -> Bus Creator/1  "Windb"
  Bus Creator/1 -> WindOut/1

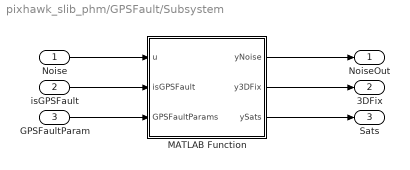
== system pixhawk_slib_phm/GPSFault/Subsystem ==
  Noise : Inport
  isGPSFault : Inport  Port=2
  GPSFaultParam : Inport  Port=3
  MATLAB Function : MATLAB Function  TreatAsAtomicUnit=on
  NoiseOut : Outport
  3DFix : Outport  Port=2
  Sats : Outport  Port=3
  wires:
  GPSFaultParam/1 -> MATLAB Function/3(GPSFaultParams)
  isGPSFault/1 -> MATLAB Function/2(isGPSFault)
  MATLAB Function/2(y3DFix) -> 3DFix/1
  MATLAB Function/3(ySats) -> Sats/1
  Noise/1 -> MATLAB Function/1(u)
  MATLAB Function/1(yNoise) -> NoiseOut/1

== system pixhawk_slib_phm/SensorFault/AccNoiseSwitch1 ==
  Noise : Inport
  isAccFault : Inport  Port=2
  AccFaultParam : Inport  Port=3
  Acc NoiseFun : MATLAB Function  TreatAsAtomicUnit=on
  NoiseOut : Outport
  wires:
  Noise/1 -> Acc NoiseFun/1(u)
  Acc NoiseFun/1(y) -> NoiseOut/1
  isAccFault/1 -> Acc NoiseFun/2(isAccFault)
  AccFaultParam/1 -> Acc NoiseFun/3(AccFaultParams)

== system pixhawk_slib_phm/SensorFault/GyroNoiseSwitch ==
  Noise : Inport
  isAccFault : Inport  Port=2
  AccFaultParam : Inport  Port=3
  Acc NoiseFun : MATLAB Function  TreatAsAtomicUnit=on
  NoiseOut : Outport
  wires:
  Noise/1 -> Acc NoiseFun/1(u)
  Acc NoiseFun/1(y) -> NoiseOut/1
  isAccFault/1 -> Acc NoiseFun/2(isAccFault)
  AccFaultParam/1 -> Acc NoiseFun/3(AccFaultParams)

== system pixhawk_slib_phm/SensorFault/GyroNoiseSwitch3 ==
  In1 : Inport
  Constant2 : Constant  Value=0.3
  Product4 : Product
  Out1 : Outport
  wires:
  Constant2/1 -> Product4/2
  Product4/1 -> Out1/1
  In1/1 -> Product4/1

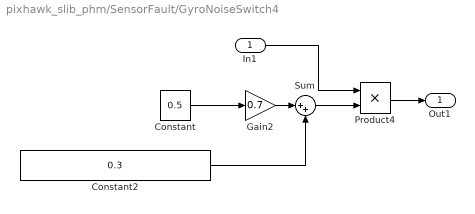
== system pixhawk_slib_phm/SensorFault/GyroNoiseSwitch4 ==
  In1 : Inport
  Constant : Constant  Value=0.5
  Constant2 : Constant  Value=0.3
  Gain2 : Gain  Gain=0.7
  Product4 : Product
  Sum : Sum  Inputs=|++
  Out1 : Outport
  wires:
  Sum/1 -> Product4/2
  Product4/1 -> Out1/1
  Gain2/1 -> Sum/1
  In1/1 -> Product4/1
  Constant2/1 -> Sum/2
  Constant/1 -> Gain2/1

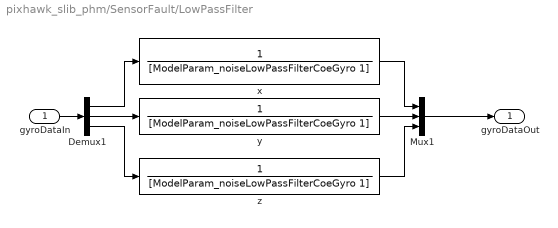
== system pixhawk_slib_phm/SensorFault/LowPassFilter ==
  gyroDataIn : Inport
  Demux1 : Demux  Outputs=3
  Mux1 : Mux  Inputs=3
  x : TransferFcn  Denominator=[ModelParam_noiseLowPassFilterCoeGyro 1]
  y : TransferFcn  Denominator=[ModelParam_noiseLowPassFilterCoeGyro 1]
  z : TransferFcn  Denominator=[ModelParam_noiseLowPassFilterCoeGyro 1]
  gyroDataOut : Outport
  wires:
  Mux1/1 -> gyroDataOut/1
  z/1 -> Mux1/3
  x/1 -> Mux1/1
  Demux1/1 -> x/1
  y/1 -> Mux1/2
  gyroDataIn/1 -> Demux1/1
  Demux1/2 -> y/1
  Demux1/3 -> z/1

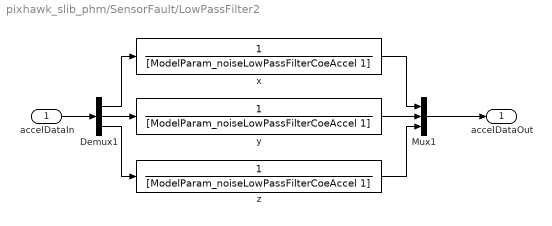
== system pixhawk_slib_phm/SensorFault/LowPassFilter2 ==
  accelDataIn : Inport
  Demux1 : Demux  Outputs=3
  Mux1 : Mux  Inputs=3
  x : TransferFcn  Denominator=[ModelParam_noiseLowPassFilterCoeAccel 1]
  y : TransferFcn  Denominator=[ModelParam_noiseLowPassFilterCoeAccel 1]
  z : TransferFcn  Denominator=[ModelParam_noiseLowPassFilterCoeAccel 1]
  accelDataOut : Outport
  wires:
  Mux1/1 -> accelDataOut/1
  z/1 -> Mux1/3
  x/1 -> Mux1/1
  Demux1/1 -> x/1
  y/1 -> Mux1/2
  accelDataIn/1 -> Demux1/1
  Demux1/2 -> y/1
  Demux1/3 -> z/1

== system pixhawk_slib_phm/SensorFault/MagNoiseSwitch ==
  Noise : Inport
  isAccFault : Inport  Port=2
  AccFaultParam : Inport  Port=3
  Acc NoiseFun : MATLAB Function  TreatAsAtomicUnit=on
  NoiseOut : Outport
  wires:
  Noise/1 -> Acc NoiseFun/1(u)
  Acc NoiseFun/1(y) -> NoiseOut/1
  isAccFault/1 -> Acc NoiseFun/2(isAccFault)
  AccFaultParam/1 -> Acc NoiseFun/3(AccFaultParams)

== system pixhawk_slib_phm/SensorFault/NoiseFilter ==
  In1 : Inport
  Demux : Demux  Outputs=3
  Mux1 : Mux  Inputs=3
  Transfer Fcn4 : TransferFcn  Denominator=[0.04 1]
  Transfer Fcn5 : TransferFcn  Denominator=[0.04 1]
  Transfer Fcn6 : TransferFcn  Denominator=[0.04 1]
  Out1 : Outport
  wires:
  Mux1/1 -> Out1/1
  In1/1 -> Demux/1
  Demux/3 -> Transfer Fcn6/1
  Transfer Fcn4/1 -> Mux1/1
  Transfer Fcn6/1 -> Mux1/3
  Demux/1 -> Transfer Fcn4/1
  Transfer Fcn5/1 -> Mux1/2
  Demux/2 -> Transfer Fcn5/1

== system pixhawk_slib_phm/SensorFault/NoiseFilter1 ==
  In1 : Inport
  Demux : Demux  Outputs=3
  Mux1 : Mux  Inputs=3
  Transfer Fcn4 : TransferFcn  Denominator=[0.04 1]
  Transfer Fcn5 : TransferFcn  Denominator=[0.04 1]
  Transfer Fcn6 : TransferFcn  Denominator=[0.04 1]
  Out1 : Outport
  wires:
  Mux1/1 -> Out1/1
  In1/1 -> Demux/1
  Demux/3 -> Transfer Fcn6/1
  Transfer Fcn4/1 -> Mux1/1
  Transfer Fcn6/1 -> Mux1/3
  Demux/1 -> Transfer Fcn4/1
  Transfer Fcn5/1 -> Mux1/2
  Demux/2 -> Transfer Fcn5/1

== system pixhawk_slib_phm/SensorFault/NoiseFilter2 ==
  In1 : Inport
  Demux : Demux  Outputs=3
  Mux1 : Mux  Inputs=3
  Transfer Fcn4 : TransferFcn  Denominator=[0.05 1]
  Transfer Fcn5 : TransferFcn  Denominator=[0.05 1]
  Transfer Fcn6 : TransferFcn  Denominator=[0.05 1]
  Out1 : Outport
  wires:
  Mux1/1 -> Out1/1
  In1/1 -> Demux/1
  Demux/3 -> Transfer Fcn6/1
  Transfer Fcn4/1 -> Mux1/1
  Transfer Fcn6/1 -> Mux1/3
  Demux/1 -> Transfer Fcn4/1
  Transfer Fcn5/1 -> Mux1/2
  Demux/2 -> Transfer Fcn5/1

== matlab function pixhawk_slib_phm/MotorFault/FaultParamsExtract1 ==
  settings: updateMethod=DISCRETE
  data: FaultID input; inInts input; hasFault output; inFloats input; FaultParam output
function [hasFault, FaultParam] = fcn(FaultID,inInts,inFloats)
persistent hFault;
persistent fParam;

if isempty(hFault)
    hFault=false;
end
if isempty(fParam)
    fParam=zeros(20,1);
end

hFaultTmp=false;
fParamTmp=zeros(20,1);
j=1;
for i=1:8
    if inInts(i) == FaultID
        hFaultTmp=true;
        fParamTmp(2*j-1)=inFloats(2*i-1);
        fParamTmp(2*j)=inFloats(2*i);
        j=j+1;
    end
end
if hFaultTmp
    hFault=hFaultTmp;
    fParamTmp(17:20) = inFloats(17:20);
    fParam=fParamTmp;
end

hasFault=hFault;
FaultParam=fParam;

== matlab function pixhawk_slib_phm/MotorFault/MotorFaultModel1 ==
  settings: updateMethod=DISCRETE
  data: hasFault input; y output; FaultParams input; inPWMs input; motNum input; noise input
function y = fcn(hasFault, FaultParams, inPWMs, motNum, noise)
% 本模块需要用到8维FaultParam的输入
%因此故障ID的格式应该是：
%inSILInts=[FaultID FaultID FaultID FaultID ...]
%inSILInts=[param1 param2 param3 param4 param5 param6 param7 param8 ...] -> FaultParam
% param的每一位表示本电机的健康系数（0到1），实际上就是pwm_out = pwm_in * param
% 如果param1=0，则电机1直接坏掉，始终输出0

y=inPWMs; %默认情况下不注入故障，直接将数据输出

if motNum<1
    motNum=int32(1);
end

if motNum>8
    motNum=int32(8);
end

if hasFault %如果注入了故障
    for i=1:motNum
        y(i) = inPWMs(i)+ FaultParams(i)*noise;
    end
end

== matlab function pixhawk_slib_phm/MotorFault/MATLAB Function ==
  data: y output; ID2 input; u1 input; u2 input
function y = fcn(ID2,u1,u2)
y=u1;
if ID2
    y=u2;
end

== matlab function pixhawk_slib_phm/SensorFault/FaultParamsExtract4 ==
  settings: updateMethod=DISCRETE
  data: FaultID input; inInts input; hasFault_accBais output; inFloats input; FaultParam output
function [hasFault_accBais, FaultParam] = fcn(FaultID,inInts,inFloats)
persistent hFault;
persistent fParam;

if isempty(hFault)
    hFault=false;
end
if isempty(fParam)
    fParam=zeros(20,1);
end

hFaultTmp=false;
fParamTmp=zeros(20,1);
j=1;
for i=1:8
    if inInts(i) == FaultID
        hFaultTmp=true;
        fParamTmp(2*j-1)=inFloats(2*i-1);
        fParamTmp(2*j)=inFloats(2*i);
        j=j+1;
    end
end
if hFaultTmp
    hFault=hFaultTmp;
    fParamTmp(17:20) = inFloats(17:20);
    fParam=fParamTmp;
end

hasFault_accBais=hFault;
FaultParam=fParam;

== matlab function pixhawk_slib_phm/GPSFault/Subsystem/MATLAB Function ==
  data: u input; yNoise output; isGPSFault input; GPSFaultParams input; y3DFix output; ySats output
function [yNoise,y3DFix,ySats] = fcn(u,isGPSFault,GPSFaultParams)

yNoise = u;
y3DFix = 3;
ySats = 10;

if isGPSFault
    yNoise = (GPSFaultParams(1))*u;
    y3DFix = GPSFaultParams(2);
    ySats = GPSFaultParams(3);
end

== matlab function pixhawk_slib_phm/GPSFault/FaultParamsExtract ==
  settings: updateMethod=DISCRETE
  data: FaultID input; inInts input; hasFault output; inFloats input; FaultParam output
function [hasFault, FaultParam] = fcn(FaultID,inInts,inFloats)
persistent hFault;
persistent fParam;

if isempty(hFault)
    hFault=false;
end
if isempty(fParam)
    fParam=zeros(20,1);
end

hFaultTmp=false;
fParamTmp=zeros(20,1);
j=1;
for i=1:8
    if inInts(i) == FaultID
        hFaultTmp=true;
        fParamTmp(2*j-1)=inFloats(2*i-1);
        fParamTmp(2*j)=inFloats(2*i);
        j=j+1;
    end
end
if hFaultTmp
    hFault=hFaultTmp;
    fParamTmp(17:20) = inFloats(17:20);
    fParam=fParamTmp;
end

hasFault=hFault;
FaultParam=fParam;

== matlab function pixhawk_slib_phm/SensorFault/baro NoiseFun1 ==
  data: isaccBaisFault input; y output; accbaisFaultParam input
function y = fcn(isaccBaisFault,accbaisFaultParam)

y = [0 0 0];
if isaccBaisFault
    for i = 1:3
        y(i) = accbaisFaultParam(i);
    end
end

== matlab function pixhawk_slib_phm/SensorFault/FaultParamsExtract ==
  settings: updateMethod=DISCRETE
  data: FaultID input; inInts input; hasFault_acc output; inFloats input; FaultParam output
function [hasFault_acc, FaultParam] = fcn(FaultID,inInts,inFloats)
persistent hFault;
persistent fParam;

if isempty(hFault)
    hFault=false;
end
if isempty(fParam)
    fParam=zeros(20,1);
end

hFaultTmp=false;
fParamTmp=zeros(20,1);
j=1;
for i=1:8
    if inInts(i) == FaultID
        hFaultTmp=true;
        fParamTmp(2*j-1)=inFloats(2*i-1);
        fParamTmp(2*j)=inFloats(2*i);
        j=j+1;
    end
end
if hFaultTmp
    hFault=hFaultTmp;
    fParamTmp(17:20) = inFloats(17:20);
    fParam=fParamTmp;
end

hasFault_acc=hFault;
FaultParam=fParam;

== matlab function pixhawk_slib_phm/SensorFault/FaultParamsExtract5 ==
  settings: updateMethod=DISCRETE
  data: FaultID input; inInts input; hasFault_gyroBais output; inFloats input; FaultParam output
function [hasFault_gyroBais, FaultParam] = fcn(FaultID,inInts,inFloats)
persistent hFault;
persistent fParam;

if isempty(hFault)
    hFault=false;
end
if isempty(fParam)
    fParam=zeros(20,1);
end

hFaultTmp=false;
fParamTmp=zeros(20,1);
j=1;
for i=1:8
    if inInts(i) == FaultID
        hFaultTmp=true;
        fParamTmp(2*j-1)=inFloats(2*i-1);
        fParamTmp(2*j)=inFloats(2*i);
        j=j+1;
    end
end
if hFaultTmp
    hFault=hFaultTmp;
    fParamTmp(17:20) = inFloats(17:20);
    fParam=fParamTmp;
end

hasFault_gyroBais=hFault;
FaultParam=fParam;

== matlab function pixhawk_slib_phm/SensorFault/baro NoiseFun2 ==
  data: isgyroBaisFault input; y output; accbaisFaultParam input
function y = fcn(isgyroBaisFault,accbaisFaultParam)

y = [0 0 0];
if isgyroBaisFault
    for i = 1:3
        y(i) = accbaisFaultParam(i);
    end
end

== matlab function pixhawk_slib_phm/SensorFault/FaultParamsExtract1 ==
  settings: updateMethod=DISCRETE
  data: FaultID input; inInts input; hasFault_gyro output; inFloats input; FaultParam output
function [hasFault_gyro, FaultParam] = fcn(FaultID,inInts,inFloats)
persistent hFault;
persistent fParam;

if isempty(hFault)
    hFault=false;
end
if isempty(fParam)
    fParam=zeros(20,1);
end

hFaultTmp=false;
fParamTmp=zeros(20,1);
j=1;
for i=1:8
    if inInts(i) == FaultID
        hFaultTmp=true;
        fParamTmp(2*j-1)=inFloats(2*i-1);
        fParamTmp(2*j)=inFloats(2*i);
        j=j+1;
    end
end
if hFaultTmp
    hFault=hFaultTmp;
    fParamTmp(17:20) = inFloats(17:20);
    fParam=fParamTmp;
end

hasFault_gyro=hFault;
FaultParam=fParam;

== matlab function pixhawk_slib_phm/SensorFault/FaultParamsExtract6 ==
  settings: updateMethod=DISCRETE
  data: FaultID input; inInts input; hasFault_magBais output; inFloats input; FaultParam output
function [hasFault_magBais, FaultParam] = fcn(FaultID,inInts,inFloats)
persistent hFault;
persistent fParam;

if isempty(hFault)
    hFault=false;
end
if isempty(fParam)
    fParam=zeros(20,1);
end

hFaultTmp=false;
fParamTmp=zeros(20,1);
j=1;
for i=1:8
    if inInts(i) == FaultID
        hFaultTmp=true;
        fParamTmp(2*j-1)=inFloats(2*i-1);
        fParamTmp(2*j)=inFloats(2*i);
        j=j+1;
    end
end
if hFaultTmp
    hFault=hFaultTmp;
    fParamTmp(17:20) = inFloats(17:20);
    fParam=fParamTmp;
end

hasFault_magBais=hFault;
FaultParam=fParam;

== matlab function pixhawk_slib_phm/SensorFault/baro NoiseFun3 ==
  data: ismagBaisFault input; y output; accbaisFaultParam input
function y = fcn(ismagBaisFault,accbaisFaultParam)

y = [0 0 0];
if ismagBaisFault
    for i = 1:3
        y(i) = accbaisFaultParam(i);
    end
end

== matlab function pixhawk_slib_phm/WindFault/MATLAB Function ==
  settings: updateMethod=DISCRETE
  data: t input; isGustWind input; gWind output; GustWindParams input; turb input
function gWind = GustWindModel(t,isGustWind,GustWindParams,turb)

if(GustWindParams(2)<1)
    GustWindParams(2)=1;
end
timeVel=60/GustWindParams(2);

vmax=GustWindParams(1);

persistent t0;
if isempty(t0)
    t0=0;
end

persistent isInGust;
if isempty(isInGust)
    isInGust=0;
end

persistent t1;
if isempty(t1)
    t1=2;
end

persistent a;
if isempty(a)
    a=0.5;
end

persistent ang;
if isempty(ang)
    ang=pi/2;
end

persistent wlast;
if isempty(wlast)
    wlast=vmax*0.5;
end

persistent wNow;
if isempty(wNow)
    wNow=1.4*0.8*vmax;
end


if isGustWind&&isInGust<0.5
    t0=t;
    t1=timeVel*(3/4+1/2*rand(1));
    a=1/4+1/2*rand(1);
    ang=pi*2*rand(1);
    wlast=wNow;
    wNow=1.2*(rand(1)*0.5+0.5)*vmax;
    
    isInGust=1;
end

if ~isGustWind
    isInGust=0;
end

gWind=[0;0;0];

if(t<t0+t1*a)
    gWindMag=(wNow-wlast)/2*(1-cos((t-t0)/(t1*a)*pi))+wlast;
else
    gWindMag=wNow;
end

if abs(t-(t0+t1))<0.05
    rng(t*1000);
    t0=t;
    t1=timeVel*(3/4+1/2*rand(1));
    a=1/4+1/2*rand(1);
    ang=ang+0.1*pi*rand(1);
    wlast=wNow;
    wNow=1.2*(rand(1)*0.5+0.5)*vmax;
end

gWind(1)=gWindMag*cos(ang)*0.8+turb(1)*0.4;
gWind(2)=gWindMag*sin(ang)*0.8+turb(2)*0.4;
gWind(3)=turb(3)*0.4;

== matlab function pixhawk_slib_phm/WindFault/MATLAB Function1 ==
  data: wind output size=3; isConstWind input; isGustWind input; isTurbWind input; isSheerWind input; ConstWind input; GustWind input; TurbWind input; SheerWind input
function wind = WindFun(isConstWind,isGustWind,isTurbWind,isSheerWind,ConstWind,GustWind,TurbWind,SheerWind)
wind=[0;0;0];
if isConstWind
    wind=[ConstWind(1);ConstWind(2);ConstWind(3)];
elseif isGustWind
    wind=GustWind;
elseif isTurbWind
    wind=TurbWind;
elseif isSheerWind
    wind=SheerWind;
end

== matlab function pixhawk_slib_phm/MotorFault/FaultParamsExtract ==
  settings: updateMethod=DISCRETE
  data: FaultID input; inInts input; hasFault output; inFloats input; FaultParam output
function [hasFault, FaultParam] = fcn(FaultID,inInts,inFloats)
persistent hFault;
persistent fParam;

if isempty(hFault)
    hFault=false;
end
if isempty(fParam)
    fParam=zeros(20,1);
end

hFaultTmp=false;
fParamTmp=zeros(20,1);
j=1;
for i=1:8
    if inInts(i) == FaultID
        hFaultTmp=true;
        fParamTmp(2*j-1)=inFloats(2*i-1);
        fParamTmp(2*j)=inFloats(2*i);
        j=j+1;
    end
end
if hFaultTmp
    hFault=hFaultTmp;
    fParamTmp(17:20) = inFloats(17:20);
    fParam=fParamTmp;
end

hasFault=hFault;
FaultParam=fParam;

== matlab function pixhawk_slib_phm/BatteryFault/FaultParamsExtract1 ==
  settings: updateMethod=DISCRETE
  data: FaultID input; inInts input; hasFault_isPowOff output; inFloats input; FaultParam output
function [hasFault_isPowOff, FaultParam] = fcn(FaultID,inInts,inFloats)
persistent hFault;
persistent fParam;

if isempty(hFault)
    hFault=false;
end
if isempty(fParam)
    fParam=zeros(20,1);
end

hFaultTmp=false;
fParamTmp=zeros(20,1);
j=1;
for i=1:8
    if inInts(i) == FaultID
        hFaultTmp=true;
        fParamTmp(2*j-1)=inFloats(2*i-1);
        fParamTmp(2*j)=inFloats(2*i);
        j=j+1;
    end
end
if hFaultTmp
    hFault=hFaultTmp;
    fParamTmp(17:20) = inFloats(17:20);
    fParam=fParamTmp;
end

hasFault_isPowOff=hFault;
FaultParam=fParam;

== matlab function pixhawk_slib_phm/WindFault/FaultParamsExtract1 ==
  settings: updateMethod=DISCRETE
  data: FaultID input; inInts input; hasFault_GustWind output; inFloats input; FaultParam output
function [hasFault_GustWind, FaultParam] = fcn(FaultID,inInts,inFloats)
persistent hFault;
persistent fParam;

if isempty(hFault)
    hFault=false;
end
if isempty(fParam)
    fParam=zeros(20,1);
end

hFaultTmp=false;
fParamTmp=zeros(20,1);
j=1;
for i=1:8
    if inInts(i) == FaultID
        hFaultTmp=true;
        fParamTmp(2*j-1)=inFloats(2*i-1);
        fParamTmp(2*j)=inFloats(2*i);
        j=j+1;
    end
end
if hFaultTmp
    hFault=hFaultTmp;
    fParamTmp(17:20) = inFloats(17:20);
    fParam=fParamTmp;
end

hasFault_GustWind=hFault;
FaultParam=fParam;

== matlab function pixhawk_slib_phm/WindFault/FaultParamsExtract4 ==
  settings: updateMethod=DISCRETE
  data: FaultID input; inInts input; hasFault_WindNoise output; inFloats input; FaultParam output
function [hasFault_WindNoise, FaultParam] = fcn(FaultID,inInts,inFloats)
persistent hFault;
persistent fParam;

if isempty(hFault)
    hFault=false;
end
if isempty(fParam)
    fParam=zeros(20,1);
end

hFaultTmp=false;
fParamTmp=zeros(20,1);
j=1;
for i=1:8
    if inInts(i) == FaultID
        hFaultTmp=true;
        fParamTmp(2*j-1)=inFloats(2*i-1);
        fParamTmp(2*j)=inFloats(2*i);
        j=j+1;
    end
end
if hFaultTmp
    hFault=hFaultTmp;
    fParamTmp(17:20) = inFloats(17:20);
    fParam=fParamTmp;
end

hasFault_WindNoise=hFault;
FaultParam=fParam;

== matlab function pixhawk_slib_phm/SensorFault/FaultParamsExtract2 ==
  settings: updateMethod=DISCRETE
  data: FaultID input; inInts input; hasFault_mag output; inFloats input; FaultParam output
function [hasFault_mag, FaultParam] = fcn(FaultID,inInts,inFloats)
persistent hFault;
persistent fParam;

if isempty(hFault)
    hFault=false;
end
if isempty(fParam)
    fParam=zeros(20,1);
end

hFaultTmp=false;
fParamTmp=zeros(20,1);
j=1;
for i=1:8
    if inInts(i) == FaultID
        hFaultTmp=true;
        fParamTmp(2*j-1)=inFloats(2*i-1);
        fParamTmp(2*j)=inFloats(2*i);
        j=j+1;
    end
end
if hFaultTmp
    hFault=hFaultTmp;
    fParamTmp(17:20) = inFloats(17:20);
    fParam=fParamTmp;
end

hasFault_mag=hFault;
FaultParam=fParam;

== matlab function pixhawk_slib_phm/SensorFault/FaultParamsExtract3 ==
  settings: updateMethod=DISCRETE
  data: FaultID input; inInts input; hasFault_baro output; inFloats input; FaultParam output
function [hasFault_baro, FaultParam] = fcn(FaultID,inInts,inFloats)
persistent hFault;
persistent fParam;

if isempty(hFault)
    hFault=false;
end
if isempty(fParam)
    fParam=zeros(20,1);
end

hFaultTmp=false;
fParamTmp=zeros(20,1);
j=1;
for i=1:8
    if inInts(i) == FaultID
        hFaultTmp=true;
        fParamTmp(2*j-1)=inFloats(2*i-1);
        fParamTmp(2*j)=inFloats(2*i);
        j=j+1;
    end
end
if hFaultTmp
    hFault=hFaultTmp;
    fParamTmp(17:20) = inFloats(17:20);
    fParam=fParamTmp;
end

hasFault_baro=hFault;
FaultParam=fParam;

== matlab function pixhawk_slib_phm/WindFault/TurbWindStrength_Dec_Switch ==
  data: vwind input size=3; TurbWind output size=3; TurbWindParams input
function TurbWind = fcn(vwind,TurbWindParams)

TurbWind=vwind*TurbWindParams(1);

== matlab function pixhawk_slib_phm/SensorFault/AccNoiseSwitch1/Acc NoiseFun ==
  data: u input; y output; isAccFault input; AccFaultParams input
function y = fcn(u,isAccFault,AccFaultParams)

y = 0.2*u;

if isAccFault
    y = (0.2+0.8*AccFaultParams(1))*u;
end

== matlab function pixhawk_slib_phm/WindFault/SheerWindStrength_Dec_Switch ==
  data: vwind input; SheerWind output; SheerWindParams input
function SheerWind = fcn(vwind,SheerWindParams)
SheerWind=vwind*SheerWindParams(1);

== matlab function pixhawk_slib_phm/SensorFault/GyroNoiseSwitch/Acc NoiseFun ==
  data: u input; y output; isAccFault input; AccFaultParams input
function y = fcn(u,isAccFault,AccFaultParams)

y = 0.2*u;

if isAccFault
    y = (0.2+0.8*AccFaultParams(1))*u;
end

== matlab function pixhawk_slib_phm/SensorFault/MagNoiseSwitch/Acc NoiseFun ==
  data: u input; y output; isAccFault input; AccFaultParams input
function y = fcn(u,isAccFault,AccFaultParams)

y = 0.2*u;

if isAccFault
    y = (0.2+0.8*AccFaultParams(1))*u;
end
